simulink model "mode_specific_reference_selection"  (R2017b)
settings: Solver=VariableStepAuto  StartTime=0.0  StopTime=10.0  RelTol=1e-3
settings Model: Creator=ernst  LastModifiedBy=ernst
settings DataIOCC: ExternalInput=[t__, u__]  LoadExternalInput=on  SaveFormat=StructureWithTime

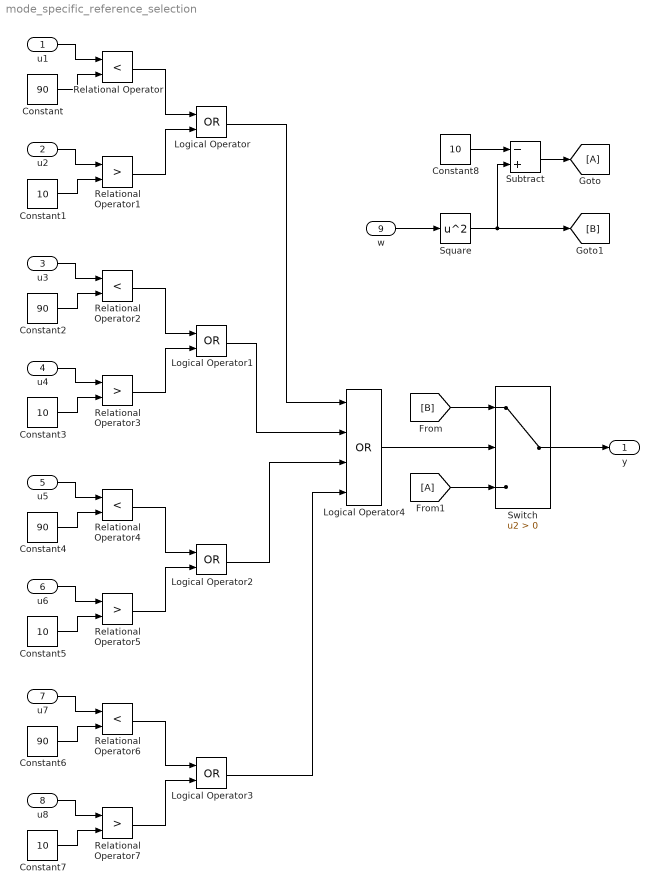
== system mode_specific_reference_selection ==
  u1 : Inport  Interpolate=off
  u2 : Inport  Port=2  Interpolate=off
  u3 : Inport  Port=3  Interpolate=off
  u4 : Inport  Port=4  Interpolate=off
  u5 : Inport  Port=5  Interpolate=off
  u6 : Inport  Port=6  Interpolate=off
  u7 : Inport  Port=7  Interpolate=off
  u8 : Inport  Port=8  Interpolate=off
  w : Inport  Port=9  Interpolate=off
  Constant{,2,4,6} (4 alike) : Constant  Value=90
  Constant{1,3,5,7..8} (5 alike) : Constant  Value=10
  Logical Operator{,1..3} (4 alike) : Logic  Operator=OR  AllPortsSameDT=off  OutDataTypeStr=boolean
  Logical Operator4 : Logic  Operator=OR  Inputs=4  AllPortsSameDT=off  OutDataTypeStr=boolean
  Relational Operator{,2,4,6} (4 alike) : RelationalOperator  Operator=<  OutDataTypeStr=boolean  RndMeth=Simplest
  Relational Operator{1,3,5,7} (4 alike) : RelationalOperator  Operator=>  OutDataTypeStr=boolean  RndMeth=Simplest
  Square : Math  Operator=square  RndMeth=Zero  SaturateOnIntegerOverflow=on
  Subtract : Sum  Inputs=-+
  Switch : Switch  Criteria=u2 > Threshold
  y : Outport
  wires:
  Switch/1 -> y/1
  [B] -> Switch/1
  [A] -> Switch/3
  u1/1 -> Relational Operator/1
  Constant/1 -> Relational Operator/2
  Relational Operator/1 -> Logical Operator/1
  u2/1 -> Relational Operator1/1
  Constant1/1 -> Relational Operator1/2
  Relational Operator1/1 -> Logical Operator/2
  Relational Operator3/1 -> Logical Operator1/2
  Constant2/1 -> Relational Operator2/2
  u4/1 -> Relational Operator3/1
  Relational Operator2/1 -> Logical Operator1/1
  Constant3/1 -> Relational Operator3/2
  u3/1 -> Relational Operator2/1
  Relational Operator5/1 -> Logical Operator2/2
  Constant4/1 -> Relational Operator4/2
  u6/1 -> Relational Operator5/1
  Relational Operator4/1 -> Logical Operator2/1
  Constant5/1 -> Relational Operator5/2
  u5/1 -> Relational Operator4/1
  Relational Operator7/1 -> Logical Operator3/2
  Constant6/1 -> Relational Operator6/2
  u8/1 -> Relational Operator7/1
  Relational Operator6/1 -> Logical Operator3/1
  Constant7/1 -> Relational Operator7/2
  u7/1 -> Relational Operator6/1
  Logical Operator4/1 -> Switch/2
  Logical Operator/1 -> Logical Operator4/1
  Logical Operator1/1 -> Logical Operator4/2
  Logical Operator2/1 -> Logical Operator4/3
  Logical Operator3/1 -> Logical Operator4/4
  w/1 -> Square/1
  Square/1 -> Subtract/2, [B]
  Subtract/1 -> [A]
  Constant8/1 -> Subtract/1
